simulink model "shifter_start"  (R2018a)
settings: Solver=FixedStepAuto  StartTime=0.0  StopTime=3.0  FixedStep=0.05  RelTol=1e-3  EnableMultiTasking=on
undefined symbols (not defined in the file): up_threshold, vehicle_speed
settings Model: Creator=jrivitus  LastModifiedBy=austi
settings DataIOCC: ExternalInput=[t, up_threshold, vehicle_speed, down_threshold ]  LimitDataPoints=on  LoadExternalInput=on  SaveFormat=Array
settings OptimizationCC: ExpressionDepthLimit=2147483647  LifeSpan=inf
settings DebuggingCC: UnderspecifiedInitializationDetection=Classic  MergeDetectMultiDrivingBlocksExec=none  ParameterPrecisionLossMsg=none  FcnCallInpInsideContextMsg=warning  AllowSymbolicDim=off  StateNameClashWarn=warning  SFUnexpectedBacktrackingDiag=warning  SFNoUnconditionalDefaultTransitionDiag=warning  SFExecutionAtInitializationDiag=none
settings HardwareCC: ProdBitPerPointer=32  ProdBitPerSizeT=32  ProdBitPerPtrDiffT=32  ProdLargestAtomicFloat=None  ProdIntDivRoundTo=Undefined  ProdEndianess=Unspecified  ProdWordSize=32  ProdHWDeviceType=32-bit Generic
settings ModelReferenceCC: PropagateSignalLabelsOutOfModel=off
settings CodeAppCC: StateflowObjectComments=on
settings GRTTargetCC: TargetLangStandard=C89/C90 (ANSI)  GeneratePreprocessorConditionals=Disable all  CombineOutputUpdateFcns=off  GRTInterface=on
settings ConfigComp: CovMetricSettings=dw  CovHtmlReporting=on  CovSaveCumulativeToWorkspaceVar=on  CovSaveSingleToWorkspaceVar=on  CovExternalEMLEnable=off  CovSFcnEnable=off

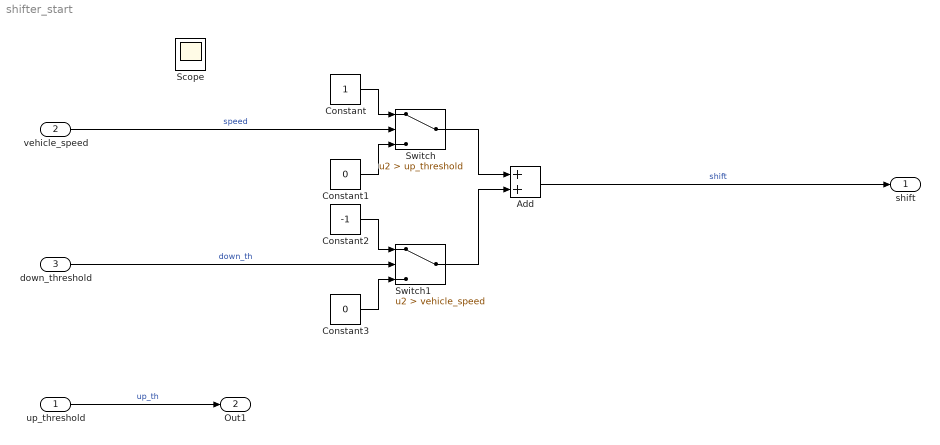
== system shifter_start ==
  up_threshold : Inport  OutDataTypeStr=double
  vehicle_speed : Inport  Port=2  OutDataTypeStr=double
  down_threshold : Inport  Port=3  OutDataTypeStr=double
  Add : Sum
  Constant : Constant
  Constant1 : Constant  Value=0
  Constant2 : Constant  Value=-1
  Constant3 : Constant  Value=0
  Switch : Switch  Criteria=u2 > Threshold  Threshold=up_threshold
  Switch1 : Switch  Criteria=u2 > Threshold  Threshold=vehicle_speed
  shift : Outport
  Out1 : Outport  Port=2
  Scope : Scope
  wires:
  up_threshold/1 -> Out1/1  "up_th"
  vehicle_speed/1 -> Switch/2  "speed"
  down_threshold/1 -> Switch1/2  "down_th"
  Add/1 -> shift/1  "shift"
  Constant1/1 -> Switch/3
  Constant3/1 -> Switch1/3
  Constant2/1 -> Switch1/1
  Switch1/1 -> Add/2
  Switch/1 -> Add/1
  Constant/1 -> Switch/1
